simulink model "DC_Motor_Push_Button_ON_OFF"  (R2024a)
settings: Solver=FixedStepDiscrete  StartTime=0.0  StopTime=inf  FixedStep=1e-3  RelTol=1e-3  EnableMultiTasking=on
libraries: arduinolib x2
settings Model: ExtModeTrigDuration=2  Creator=DELL  LastModifiedBy=DELL
settings SolverCC: AutoInsertRateTranBlk=on
settings OptimizationCC: EnhancedBackFolding=on  PassReuseOutputArgsAs=Individual arguments  ZeroExternalMemoryAtStartup=off  ZeroInternalMemoryAtStartup=off  MaxStackSize=64  OptimizeBlockOrder=speed  DifferentSizesBufferReuse=on  OptimizationCustomize=off  EfficientTunableParamExpr=on
settings DebuggingCC: ParameterTunabilityLossMsg=error
settings HardwareCC: ProdBitPerInt=16  ProdBitPerPointer=16  ProdBitPerSizeT=16  ProdBitPerPtrDiffT=16  ProdLargestAtomicFloat=None  ProdWordSize=8  ProdHWDeviceType=Atmel->AVR
settings SFSimCC: MATLABDynamicMemAlloc=off
settings RTWCC: Description=Embedded Coder  SystemTargetFile=ert.tlc  HardwareBoard=Arduino Uno  TemplateMakefile=ert_default_tmf  Toolchain=Arduino AVR  BuildConfiguration=Faster Runs
settings CodeAppCC: ForceParamTrailComments=on  IgnoreCustomStorageClasses=off  OperatorAnnotations=on  SimulinkDataObjDesc=on  SFDataObjDesc=on  InsertBlockDesc=on
settings ERTTargetCC: SupportContinuousTime=on  SupportVariableSizeSignals=on  ExtModeTransport=3  ExtModeStaticAlloc=on  ExtModeAutomaticAllocSize=off  ExtModeStaticAllocSize=250  ExtModeMexFile=ext_xcp  ExtModeIntrfLevel=Level2 - Open

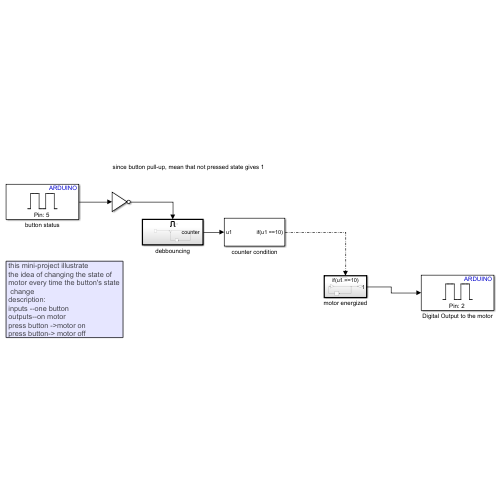
[thumbnail: Simulink's stored preview of the top-level diagram]
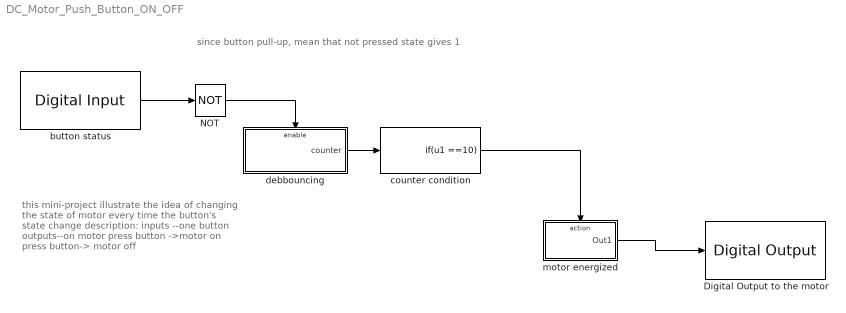
== system DC_Motor_Push_Button_ON_OFF ==
  note: this mini-project illustrate
      | the idea of changing the state of
      | motor every time the button's state
      |  change
      | description:
      | inputs --one button
      | outputs--on motor
      | press button ->motor on
      | press button-> motor off
  note: since button pull-up, mean that not pressed state gives 1
  Digital Output to the motor : arduinolib/Digital Output  pinNumber=2  Direction=output  blockPlatform=arduino
  NOT : Logic  Operator=NOT  IconShape=distinctive  AllPortsSameDT=off  OutDataTypeStr=boolean
  button status : arduinolib/Digital Input  pinNumber=5  mode=Input Pullup  Direction=input  SampleTime=0.1  blockPlatform=arduino
  counter condition : If  IfExpression=u1 ==10  ShowElse=off
  debbouncing : Subsystem  TreatAsAtomicUnit=on
  motor energized : Subsystem  TreatAsAtomicUnit=on
  wires:
  button status/1 -> NOT/1
  debbouncing/1("counter ") -> counter condition/1
  NOT/1 -> debbouncing/Enable
  motor energized/1(Out1) -> Digital Output to the motor/1
  counter condition/1 -> motor energized/Action

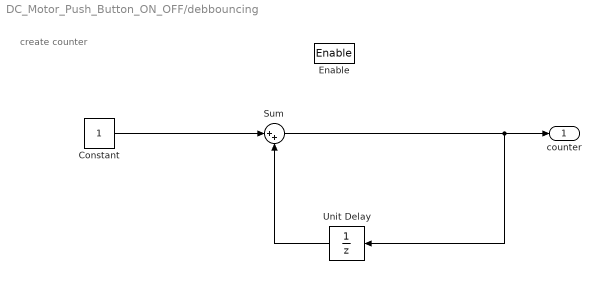
== system DC_Motor_Push_Button_ON_OFF/debbouncing ==
  note: create counter
  Enable : EnablePort  StatesWhenEnabling=reset
  Constant : Constant
  Sum : Sum  Inputs=|++
  Unit Delay : UnitDelay  SampleTime=-1  HasFrameUpgradeWarning=on
  "counter " : Outport
  wires:
  Unit Delay/1 -> Sum/2
  Sum/1 -> "counter "/1, Unit Delay/1
  Constant/1 -> Sum/1

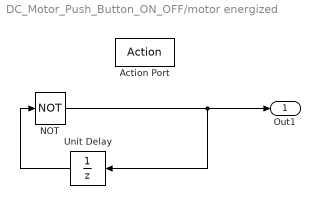
== system DC_Motor_Push_Button_ON_OFF/motor energized ==
  Action Port : ActionPort  ActionPortLabel=if(u1 ==10)
  NOT : Logic  Operator=NOT  IconShape=distinctive  AllPortsSameDT=off  OutDataTypeStr=boolean
  Unit Delay : UnitDelay  SampleTime=-1  HasFrameUpgradeWarning=on
  Out1 : Outport
  wires:
  NOT/1 -> Unit Delay/1, Out1/1
  Unit Delay/1 -> NOT/1
